simulink model "pcssp_cruise_controller"  (R2021b)
settings: configuration reference "configurationSettings" (kept outside this file)
undefined symbols (not defined in the file or in its folder): cruise_controller_fp, cruise_controller_tp
libraries: slpidlib x1
settings Model: DataDictionary=pcssp_cruise_controller.sldd  Creator=timoravensbergen  LastModifiedBy=timoravensbergen
settings ConfigSetRef: SourceName=configurationSettings

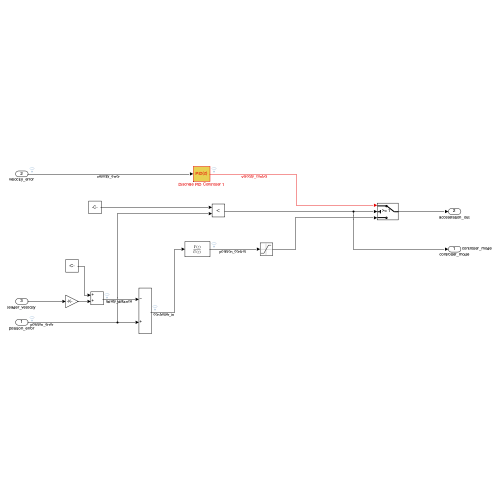
[thumbnail: Simulink's stored preview of the top-level diagram]
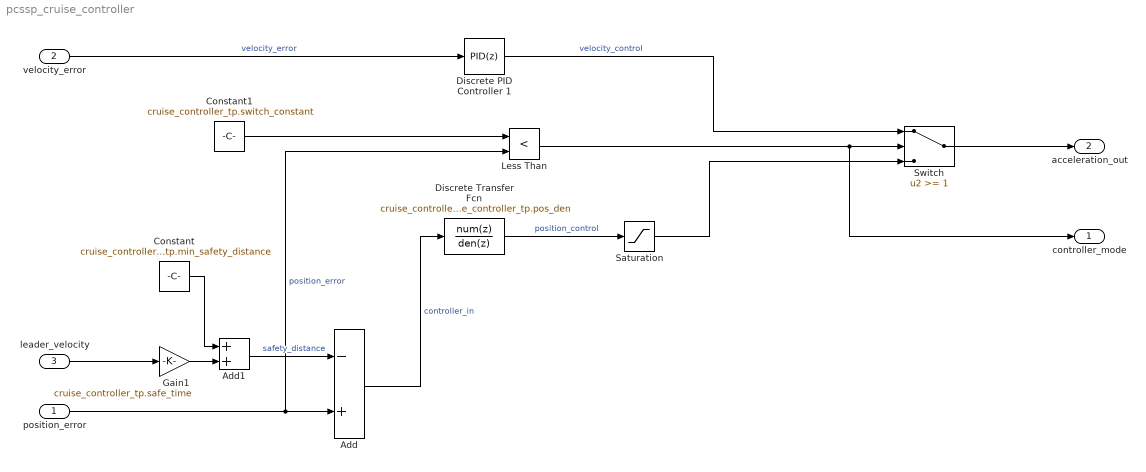
== system pcssp_cruise_controller ==
  position_error : Inport  SampleTime=cruise_controller_fp.timing.dt
  velocity_error : Inport  Port=2  SampleTime=cruise_controller_fp.timing.dt
  leader_velocity : Inport  Port=3  SampleTime=cruise_controller_fp.timing.dt
  Add : Sum  Inputs=-+
  Add1 : Sum
  Constant : Constant  Value=cruise_controller_tp.min_safety_distance
  Constant1 : Constant  Value=cruise_controller_tp.switch_constant
  Discrete Transfer Fcn : DiscreteTransferFcn  Numerator=cruise_controller_tp.pos_num  Denominator=cruise_controller_tp.pos_den
  Discrete PID Controller 1 : slpidlib/PID Controller  Controller=PID  Form=Parallel  TimeDomain=Discrete-time  UseExternalTs=off  SampleTime=-1  IntegratorMethod=Forward Euler  FilterMethod=Forward Euler  ControllerParametersSource=internal  P=cruise_controller_tp.Pvel  I=cruise_controller_tp.Ivel  D=cruise_controller_tp.Dvel  N=100  UseFilter=on  TunerSelectOption=Transfer Function Based (PID Tuner App)  InitialConditionSource=internal  InitialConditionForIntegrator=0  InitialConditionForFilter=0  DifferentiatorICPrevScaledInput=0  ExternalReset=none  TrackingMode=off  Kt=1  LimitOutput=off  SatLimitsSource=internal  UpperSaturationLimit=inf  LowerSaturationLimit=-inf  LinearizeAsGain=off  AntiWindupMode=none  Kb=1  POutMin=[]  POutMax=[]  IOutMin=[]  IOutMax=[]  DOutMin=[]  DOutMax=[]  NOutMin=[]  NOutMax=[]  SumOutMin=[]  SumOutMax=[]  SaturationOutMin=[]  SaturationOutMax=[]  PParamMin=[]  PParamMax=[]  IParamMin=[]  IParamMax=[]  DParamMin=[]  DParamMax=[]  NParamMin=[]  NParamMax=[]  KbParamMin=[]  KbParamMax=[]  KtParamMin=[]  KtParamMax=[]  KbOutMin=[]  KbOutMax=[]  KtOutMin=[]  KtOutMax=[]  IntegratorOutMin=[]  IntegratorOutMax=[]  FilterOutMin=[]  FilterOutMax=[]  SumI1OutMin=[]  SumI1OutMax=[]  SumI2OutMin=[]  SumI2OutMax=[]  SumI3OutMin=[]  SumI3OutMax=[]  SumI4OutMin=[]  SumI4OutMax=[]  SumDOutMin=[]  SumDOutMax=[]  DifferentiatorOutMin=[]  DifferentiatorOutMax=[]  FilterDiffOutCoefMin=[]  FilterDiffOutCoefMax=[]  ReciprocalOutMin=[]  ReciprocalOutMax=[]  SumDenOutMin=[]  SumDenOutMax=[]  SumNumOutMin=[]  SumNumOutMax=[]  DivideOutMin=[]  DivideOutMax=[]  UdiffTsProdOutMin=[]  UdiffTsProdOutMax=[]  NTsProdOutMin=[]  NTsProdOutMax=[]  UintegralTsProdOutMin=[]  UintegralTsProdOutMax=[]  UngainTsProdOutMin=[]  UngainTsProdOutMax=[]  IntegratorContinuousStateAttributes=''  IntegratorStateMustResolveToSignalObject=off  IntegratorRTWStateStorageClass=Auto  FilterContinuousStateAttributes=''  FilterStateMustResolveToSignalObject=off  FilterRTWStateStorageClass=Auto  ParallelPVariant=InternalParameters  IdealPVariant=Disabled  IVariant=InternalParameters  DVariant=InternalParameters  IntegratorVariant=Discrete  SatVariant=Disabled  AWVariant=Passthrough  PCopyVariant=Disabled  TRVariant=Disabled  FdbkBlocksVariant=Forward  IdealPFdbkVariant=Disabled  SatFdbkVariant=Disabled  DerivativeFilterVariant=ForwardEulerFilter  NVariant=InternalParameters  NCopyVariant=Disabled  FilterICVariant=InternalICsFilter  IntegratorICVariant=InternalICs  ExternalResetVariant=Disabled  TRSumVariant=Passthrough  SumFdbkVariant=Disabled  SumVariant=Sum_PID  TsampFilterVariant=InternalTs  TsampNgainVariant=Passthrough  TsampIntegralVariant=Disabled_SignalSpec  ExternalSaturationOutDataTypeStr=Inherit: Same as second input
  Gain1 : Gain  Gain=cruise_controller_tp.safe_time
  Less Than : RelationalOperator  Operator=<  OutDataTypeStr=boolean  RndMeth=Simplest
  Saturation : Saturate  UpperLimit=cruise_controller_tp.pos_acc_saturation  LowerLimit=cruise_controller_tp.neg_acc_saturation
  Switch : Switch  Threshold=1
  controller_mode : Outport  SignalName=controller_mode
  acceleration_out : Outport  Port=2
  wires:
  velocity_error/1 -> Discrete PID Controller 1/1  "velocity_error"
  Discrete PID Controller 1/1 -> Switch/1  "velocity_control"
  Discrete Transfer Fcn/1 -> Saturation/1  "position_control"
  Switch/1 -> acceleration_out/1
  Less Than/1 -> controller_mode/1, Switch/2
  leader_velocity/1 -> Gain1/1
  Constant1/1 -> Less Than/1
  Saturation/1 -> Switch/3
  Add1/1 -> Add/1  "safety_distance"
  Constant/1 -> Add1/1
  Gain1/1 -> Add1/2
  Add/1 -> Discrete Transfer Fcn/1  "controller_in"
  position_error/1 -> Less Than/2, Add/2  "position_error"
